simulink model "BasicSimulink"  (R2020a)
settings: configuration reference "Configuration" (kept outside this file)
PostLoadFcn:
  | if(exist('BasicSimulink_init_DB.m','file'))
  | BasicSimulink_init_DB
  | else
  | BasicSimulink_init
  | end
values from neighbouring files (symbols this model uses):
  Sim = genTurbineModelParameters(simParam,modelData)    [BasicSimulink_init.m]
undefined symbols (not defined in the file or in its folder): Const, ControllerState, OpMode
libraries: CustomBlocks_lib x1, TurbinePhysics_lib x1
settings Model: Creator=12650008  LastModifiedBy=80679
settings ConfigSetRef: SourceName=Configuration  SourceLocation=Base Workspace

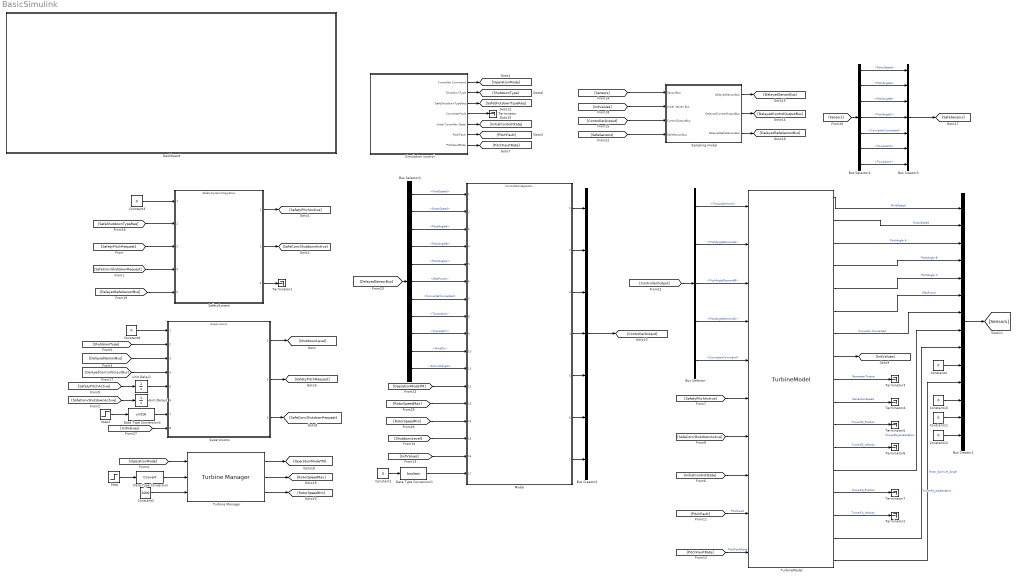
== system BasicSimulink ==
  Bus Creator1 : BusCreator  Inputs=14  OutDataTypeStr=Bus: SensorBus  NonVirtualBus=on
      settings: InheritFromInputs=off
  Bus Creator2 : BusCreator  Inputs=7  OutDataTypeStr=Bus: ControllerOutputBus  NonVirtualBus=on
      settings: InheritFromInputs=off
  Bus Creator3 : BusCreator  Inputs=7  OutDataTypeStr=Bus: SafeSensorBus  NonVirtualBus=on
      settings: InheritFromInputs=off
  Bus Selector : BusSelector  OutputSignals=TorqueDemand,PitchAngleDemandA,PitchAngleDemandB,PitchAngleDemandC,ConverterCommand
  Bus Selector1 : BusSelector  OutputSignals=WindSpeed,RotorSpeed,PitchAngleA,PitchAngleB,PitchAngleC,ElecPower,ConverterConnected,TowerAccX,TowerAccY,WindDir,AzimuthAngle
  Bus Selector2 : BusSelector  OutputSignals=RotorSpeed,PitchAngleA,PitchAngleB,PitchAngleC,ConverterConnected,TowerAccX,TowerAccY
  Constant1 : Constant  Value=0  OutDataTypeStr=boolean
  Constant{4,10..12} (4 alike) : Constant  Value=0
  Constant2 : Constant  Value=1000  OutDataTypeStr=uint16
  Constant3 : Constant  Value=0  OutDataTypeStr=boolean
  Constant6 : Constant  Value=0  OutDataTypeStr=boolean
  Dashboard : Subsystem
  Data Type Conversion : DataTypeConversion
  Data Type Conversion1 : DataTypeConversion  OutDataTypeStr=boolean
  Data Type Conversion3 : DataTypeConversion  OutDataTypeStr=uint16
  Model : ModelReference  ModelNameDialog=ControllerIntegration.slx  SimulationMode=Normal  ModelReferenceVersion=1.784
  SafetySystem : ModelReference  ModelNameDialog=SafetySystemIntegration.slx  SimulationMode=Normal  ModelReferenceVersion=1.139
  Sampling model : Subsystem
  Simulation control : Subsystem  mask{SimCase=1, VarType=NormalProduction}
      mask prompts: SimCase "Case"; VarType "Simulink:Variants:LabelComboBox"
      mask init:
      | switch (SimCase)
      |     case 1
      |         set_param(gcbh,'VarType','NormalProduction');
      |     case 2
      |         set_param(gcbh,'VarType','Startup');
      |     case 3
      |         set_param(gcbh,'VarType','Shutdown');
      |     case 4
      |         set_param(gcbh,'VarType','NoPitch');
      |     case 5
      |         set_param(gcbh,'VarType','NoTorque');
      |     case 6
      |         set_param(gcbh,'VarType','SafetySystem');
      |     case 7
      |         set_param(gcbh,'VarType','PitchRunaway');
      | end
      mask TypeOptions VarType: Scenario control/LabelModeActiveChoice
      mask DialogControl VarType Prompt: Label mode active choice:
  Step : Step  Time=3000  After=0  SampleTime=Const.Ts
  Step2 : Step  Time=30  Before=32  After=0  SampleTime=Const.Ts
  Supervisions : ModelReference  ModelNameDialog=Supervisions.slx  SimulationMode=Normal  ModelReferenceVersion=1.118
  Terminator{,1..7} (8 alike) : Terminator
  Turbine Manager : CustomBlocks_lib/Turbine Manager  SystemSampleTime=-1  Latency=0  AutoFrameSizeCalculation=off
      settings: SourceProductName=SEWPG Library
  TurbineModel : TurbinePhysics_lib/TurbineModel  Ts=Const.Ts  SimCase=6  RotAzimuthInit=0  EnableTurbulence=0  ScaleTurbulence=0.5  Seed=315  WindSpdMean=25  MeanShape=3  SineAmplitude=6  SineFrequency=0.01  RampSlope=0.01  RotorDiameter=Sim.RotorDiameter  AirDensity=Sim.AirDensity  CpData=Sim.Cp_data  CpTSR=Sim.Cp_TSR  CpPitch=Sim.Cp_pitch  dCpData=Sim.dCpdBeta  CtData=Sim.Ct_data  CtTSR=Sim.Ct_TSR  CtPitch=Sim.Ct_pitch  MaxPitch=Sim.MaxPitch  MinPitch=Sim.MinPitch  P_term=Sim.PitchSpeedGain  Acc_LimitUpper=Sim.PitchAccRateMax  Acc_LimitLower=Sim.PitchAccRateMin  MaxPitchRate=Sim.PitchModelRamp  PitchTau=Sim.PitchTau  InitialPitch=Sim.InitialPitch  PitchDelay=Sim.PitchModelDelay  SafetyPitchRate=Sim.SafetyPitchRate  Inertia=Sim.Inertia  GearRatio=Sim.GearRatio  FrictionOffset=Sim.FrictionOffset  FrictionGain=Sim.FrictionGain  DriveTrainModelSelector=Sim.DriveTrainModelSelector  MechLossTorqBp=Sim.MechLoss.TorqueBp  MechLossSpdBp=Sim.MechLoss.SpdBp  MechLossData=Sim.MechLoss.Table  BladedMechLossBp=Sim.BladedMechLossBp  BladedMechLoss=Sim.BladedMechLoss  ConverterTimeConstant=Sim.ConverterTimeConstant  ConverterConnectDelay=Sim.ConverterConnectDelay  DecayTime=Sim.ConverterDecayTime  K_comp=Sim.K_LossCompGain  LossCompMinRotSpdFactor=Sim.LossCompMinRotSpdFactor  minRotSpd=Sim.RotorSpdMin  ElEffData=Sim.ElecEff.Table  EllEffSpeedBp=Sim.ElecEff.SpdBp  ElEffPowBp=Sim.ElecEff.PowBp  BladedElecLoss=Sim.BladedElecLoss  BladedElecLossBp=Sim.BladedElecLossBp  OwnConsData=Sim.OwnCons.Table  OwnConsSpeedBp=Sim.OwnCons.SpdBp  MaxTorqueSpdSlope=Sim.MaxTorqueSpdSlope  MaxTorqueLim=Sim.MaxTorqueLim  MinTorqueSpdSlope=Sim.MinTorqueSpdSlope  MinTorqueLim=Sim.MinTorqueLim  MaxSpeedLim=Sim.MaxSpeedLim  RotorSpeedFiltFreq=Sim.RotorSpeedFiltFreq  EnableTorqueSpeedLimit=Sim.EnableTorqueSpeedLimit  twrFirstModeMass=Sim.twr.FirstModeMass  twrFirstModeLogDec=Sim.twr.FirstModeLogDec  twrFirstModeFrequencyHz=Sim.twr.FirstModeFrequencyHz  twrHeight=Sim.twr.Height
      settings: SourceProductName=SEWPG Library
  Unit Delay1 : UnitDelay  SampleTime=-1  HasFrameUpgradeWarning=on
  Unit Delay2 : UnitDelay  SampleTime=-1  HasFrameUpgradeWarning=on
  wires:
  TurbineModel/7 -> Bus Creator1/7  "Conveter Connected"
  TurbineModel/8 -> [InitValues]
  Simulation control/1(Controller Command) -> [OperationMode]
  Simulation control/2(ShutdownType) -> [ShutdownType]
  Simulation control/5(Initial Controller State) -> [InitialControlState]
  [InitialControlState] -> TurbineModel/8
  [SafetyPitchActive] -> TurbineModel/6
  [SafeConvShutdownActive] -> TurbineModel/7
  TurbineModel/9 -> Terminator3/1  "GeneratorTorque"
  TurbineModel/10 -> Terminator4/1  "GeneratorSpeed"
  TurbineModel/11 -> Terminator5/1  "TowerSS_Position"
  TurbineModel/12 -> Terminator6/1  "TowerSS_Velocity"
  [ShutdownType] -> Supervisions/2
  Constant6/1 -> Supervisions/1
  Bus Creator1/1 -> [Sensors]
  Bus Creator2/1 -> [ControllerOutput]
  [DelayedControlOutputBus] -> Supervisions/4
  Unit Delay1/1 -> Supervisions/5
  Unit Delay2/1 -> Supervisions/6
  [ControllerOutput] -> Bus Selector/1
  Bus Selector/1 -> TurbineModel/1  "<TorqueDemand>"
  Bus Selector/2 -> TurbineModel/2  "<PitchAngleDemandA>"
  Bus Selector/5 -> TurbineModel/5  "<ConverterCommand>"
  TurbineModel/1 -> Bus Creator1/1  "WindSpeed"
  TurbineModel/2 -> Bus Creator1/2  "RotorSpeed"
  TurbineModel/6 -> Bus Creator1/6  "ElecPower"
  Supervisions/3 -> [SafeConvShutdownRequest]
  Supervisions/2 -> [SafetyPitchRequest]
  SafetySystem/1 -> [SafetyPitchActive]
  SafetySystem/2 -> [SafeConvShutdownActive]
  [SafeConvShutdownActive] -> Unit Delay2/1
  [SafetyPitchActive] -> Unit Delay1/1
  Supervisions/1 -> [ShutdownLevel]
  [PitchFault] -> TurbineModel/9  "PitchFault"
  [PitchFaultRate] -> TurbineModel/10  "PitchFaultRate"
  Simulation control/6(PitchFault) -> [PitchFault]
  Simulation control/7(PitchFaultRate) -> [PitchFaultRate]
  Constant3/1 -> SafetySystem/1
  [SafeConvShutdownRequest] -> SafetySystem/4
  [SafetyPitchRequest] -> SafetySystem/3
  Simulation control/4(ConverterFault) -> Terminator/1
  Simulation control/3(SafeShutdownTypeReq) -> [SafeShutdownTypeReq]
  [SafeShutdownTypeReq] -> SafetySystem/2
  SafetySystem/3 -> Terminator1/1
  [DelayedSensorBus] -> Supervisions/3
  [DelayedSensorBus] -> Bus Selector1/1
  [Sensors] -> Sampling model/1(SensorBus)
  [InitValues] -> Sampling model/2(Initial Values Bus)
  [ControllerOutput] -> Sampling model/3(ControlOutputBus)
  Sampling model/1(DelayedSensorBus) -> [DelayedSensorBus]
  Sampling model/2(DelayedControlOutputBus) -> [DelayedControlOutputBus]
  TurbineModel/13 -> Bus Creator1/8  "TowerSS_acceleration"
  Bus Creator3/1 -> [SafeSensors]
  Bus Selector2/7 -> Bus Creator3/7  "<TowerAccY>"
  Bus Selector2/6 -> Bus Creator3/6  "<TowerAccX>"
  Bus Selector2/5 -> Bus Creator3/5  "<ConverterConnected>"
  Bus Selector2/4 -> Bus Creator3/4  "<PitchAngleC>"
  Bus Selector2/3 -> Bus Creator3/3  "<PitchAngleB>"
  Bus Selector2/2 -> Bus Creator3/2  "<PitchAngleA>"
  Bus Selector2/1 -> Bus Creator3/1  "<RotorSpeed>"
  [DelayedSafeSensorBus] -> SafetySystem/5
  [Sensors] -> Bus Selector2/1
  [SafeSensors] -> Sampling model/4(SafeSensorBus)
  Sampling model/3(DelayedSafeSensorBus) -> [DelayedSafeSensorBus]
  Step/1 -> Data Type Conversion/1
  Turbine Manager/1 -> [OperationModeTM]
  Turbine Manager/2 -> [RotorSpeedMax]
  Turbine Manager/3 -> [RotorSpeedMin]
  Data Type Conversion/1 -> Turbine Manager/2
  Step2/1 -> Data Type Conversion3/1
  Constant2/1 -> Turbine Manager/3
  Model/1 -> Bus Creator2/1
  Model/2 -> Bus Creator2/2
  Model/3 -> Bus Creator2/3
  Model/4 -> Bus Creator2/4
  Model/5 -> Bus Creator2/5
  Model/6 -> Bus Creator2/6
  Model/7 -> Bus Creator2/7
  [InitValues] -> Model/16
  [ShutdownLevel] -> Model/15
  [RotorSpeedMin] -> Model/14
  [OperationModeTM] -> Model/12
  [RotorSpeedMax] -> Model/13
  Constant12/1 -> Bus Creator1/14
  Constant11/1 -> Bus Creator1/13
  Constant10/1 -> Bus Creator1/12
  Data Type Conversion3/1 -> Supervisions/7
  [InitValues] -> Supervisions/8
  [OperationMode] -> Turbine Manager/1
  Constant1/1 -> Data Type Conversion1/1
  Data Type Conversion1/1 -> Model/17
  TurbineModel/14 -> Terminator7/1  "TowerFA_Position"
  TurbineModel/15 -> Terminator2/1  "TowerFA_Velocity"
  TurbineModel/16 -> Bus Creator1/9  "TowerFA_acceleration"
  TurbineModel/17 -> Bus Creator1/11  "Rotor_Azimuth_Angle"
  Constant4/1 -> Bus Creator1/10
  Bus Selector/3 -> TurbineModel/3  "<PitchAngleDemandB>"
  Bus Selector/4 -> TurbineModel/4  "<PitchAngleDemandC>"
  TurbineModel/3 -> Bus Creator1/3  "PitchAngle A"
  TurbineModel/4 -> Bus Creator1/4  "PitchAngle B"
  TurbineModel/5 -> Bus Creator1/5  "PitchAngle C"
  Bus Selector1/1 -> Model/1  "<WindSpeed>"
  Bus Selector1/2 -> Model/2  "<RotorSpeed>"
  Bus Selector1/3 -> Model/3  "<PitchAngleA>"
  Bus Selector1/4 -> Model/4  "<PitchAngleB>"
  Bus Selector1/5 -> Model/5  "<PitchAngleC>"
  Bus Selector1/6 -> Model/6  "<ElecPower>"
  Bus Selector1/7 -> Model/7  "<ConverterConnected>"
  Bus Selector1/8 -> Model/8  "<TowerAccX>"
  Bus Selector1/9 -> Model/9  "<TowerAccY>"
  Bus Selector1/10 -> Model/10  "<WindDir>"
  Bus Selector1/11 -> Model/11  "<AzimuthAngle>"

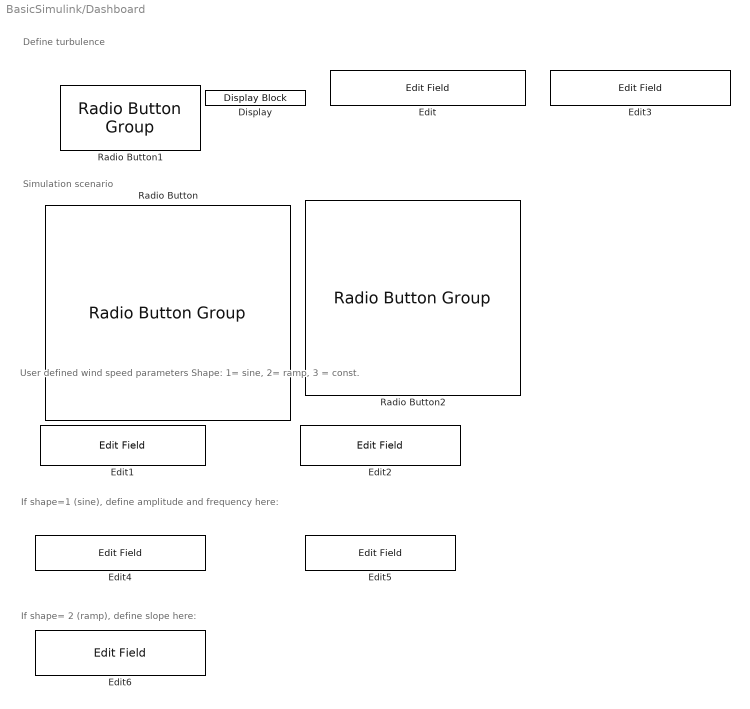
== system BasicSimulink/Dashboard ==
  note: Simulation scenario
  note: Define turbulence
  note: If shape= 2 (ramp), define slope here:
  note: If shape=1 (sine), define amplitude and frequency here:
  note: User defined wind speed parameters
      | Shape: 1= sine, 2= ramp, 3 = const.
  Display : DisplayBlock  LabelPosition=Hide  Format=Custom  Transparency=1  Layout=Fill available space  FormatString=Simulation time: %d
  Edit{,1..6} (7 alike) : EditField  ShowInitialText=on  Alignment=Center
  Radio Button : RadioButtonGroup  LabelPosition=Hide  SelectedLabel=6: User defined by parameters  ButtonGroupName=Wind Speed Control
      settings: Values={{'1: Low Wind', '2: Medium Wind', '3: High Wind', '4: Ramp mean wind speed', '5: Sinusoidal Wind Speed', '6: User defined by parameters'}, [1 2 3 4 5 6]}
  Radio Button1 : RadioButtonGroup  LabelPosition=Hide  SelectedLabel=Disabled  ButtonGroupName=Turbulence
      settings: Values={{'Disabled', 'Enabled'}, [0 1]}
  Radio Button2 : RadioButtonGroup  LabelPosition=Hide  SelectedLabel=Normal Production  ButtonGroupName=Simulation Control
      settings: Values={{'Normal Production', 'Startup', 'Shutdown (normal)', 'Shutdown (PitchFault)', 'Shutdown (Converter fault)', 'Shutdown (SafetySystem)', 'PitchRunaway'}, [1 2 3 4 5 6 7]}

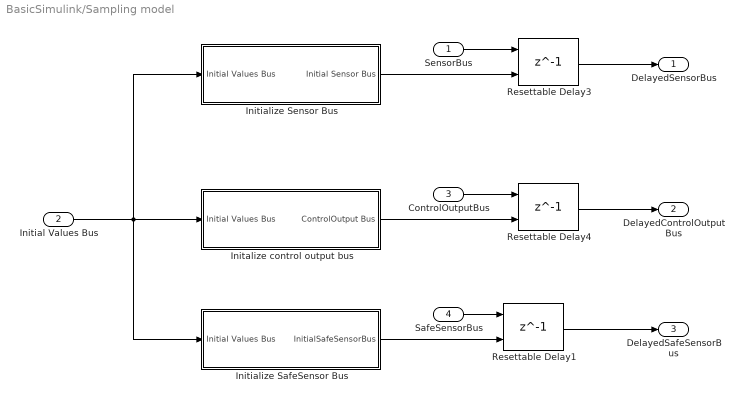
== system BasicSimulink/Sampling model ==
  SensorBus : Inport
  Initial Values Bus : Inport  Port=2
  ControlOutputBus : Inport  Port=3
  SafeSensorBus : Inport  Port=4
  Initalize control output bus : Subsystem  mask{gearratio=Sim.GearRatio}
      mask prompts: gearratio "Gear ratio"
      mask TypeOptions gearratio: GearRatio/Value
  Initialize SafeSensor Bus : Subsystem
  Initialize Sensor Bus : Subsystem
  Resettable Delay1 : Delay  DelayLength=1  InitialConditionSource=Input port  SampleTime=Const.Ts
      settings: InputPortMap=u0,p4
  Resettable Delay3 : Delay  DelayLength=1  InitialConditionSource=Input port  SampleTime=Const.Ts
      settings: InputPortMap=u0,p4
  Resettable Delay4 : Delay  DelayLength=1  InitialConditionSource=Input port  SampleTime=Const.Ts
      settings: InputPortMap=u0,p4
  DelayedSensorBus : Outport
  DelayedControlOutputBus : Outport  Port=2
  DelayedSafeSensorBus : Outport  Port=3
  wires:
  Initalize control output bus/1(ControlOutput Bus) -> Resettable Delay4/2
  Initialize Sensor Bus/1(Initial Sensor Bus) -> Resettable Delay3/2
  Resettable Delay4/1 -> DelayedControlOutputBus/1
  ControlOutputBus/1 -> Resettable Delay4/1
  Resettable Delay3/1 -> DelayedSensorBus/1
  SensorBus/1 -> Resettable Delay3/1
  Initial Values Bus/1 -> Initalize control output bus/1(Initial Values Bus), Initialize SafeSensor Bus/1(Initial Values Bus), Initialize Sensor Bus/1(Initial Values Bus)
  Initialize SafeSensor Bus/1(InitialSafeSensorBus) -> Resettable Delay1/2
  Resettable Delay1/1 -> DelayedSafeSensorBus/1
  SafeSensorBus/1 -> Resettable Delay1/1

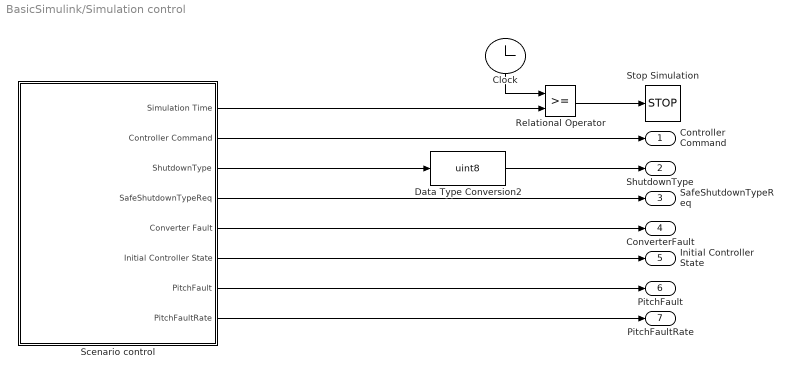
== system BasicSimulink/Simulation control ==
  Clock : Clock
  Data Type Conversion2 : DataTypeConversion  OutDataTypeStr=uint8
  Relational Operator : RelationalOperator  OutDataTypeStr=boolean  RndMeth=Simplest
  Scenario control : Subsystem  Variant=on  VariantControlMode=Label  VariantControl=Startup  LabelModeActiveChoice=NormalProduction
  Stop Simulation : Stop
  Controller Command : Outport
  ShutdownType : Outport  Port=2
  SafeShutdownTypeReq : Outport  Port=3
  ConverterFault : Outport  Port=4
  Initial Controller State : Outport  Port=5
  PitchFault : Outport  Port=6
  PitchFaultRate : Outport  Port=7
  wires:
  Clock/1 -> Relational Operator/1
  Relational Operator/1 -> Stop Simulation/1
  Scenario control/1(Simulation Time) -> Relational Operator/2
  Scenario control/4(SafeShutdownTypeReq) -> SafeShutdownTypeReq/1
  Scenario control/5(Converter Fault) -> ConverterFault/1
  Scenario control/3(ShutdownType) -> Data Type Conversion2/1
  Scenario control/6(Initial Controller State) -> Initial Controller State/1
  Scenario control/2(Controller Command) -> Controller Command/1
  Data Type Conversion2/1 -> ShutdownType/1
  Scenario control/7(PitchFault) -> PitchFault/1
  Scenario control/8(PitchFaultRate) -> PitchFaultRate/1

== system BasicSimulink/Sampling model/Initalize control output bus ==
  Initial Values Bus : Inport
  Bus Creator3 : BusCreator  Inputs=7  OutDataTypeStr=Bus: ControllerOutputBus  NonVirtualBus=on
      settings: InheritFromInputs=off
  Bus Selector2 : BusSelector  OutputSignals=RotorTorque,PitchAngle,RotorSpeed,ControllerState
  Constant : Constant  Value=ControllerState.Production  OutDataTypeStr=Enum: ControllerState
  Constant1 : Constant  Value=ControllerState.Production  OutDataTypeStr=Enum: ControllerState
  Data Type Conversion : DataTypeConversion  OutDataTypeStr=uint8
  Divide : Product  Inputs=*/
  GearRatio : Constant  Value=gearratio
  Relational Operator : RelationalOperator  Operator===  OutDataTypeStr=boolean  RndMeth=Nearest
  ControlOutput Bus : Outport
  wires:
  Bus Selector2/3 -> Bus Creator3/6  "<RotorSpeed>"
  Bus Selector2/2 -> Bus Creator3/5, Bus Creator3/4, Bus Creator3/3  "<PitchAngle>"
  Divide/1 -> Bus Creator3/2  "InitGenTorque"
  Bus Selector2/1 -> Divide/1  "<RotorTorque>"
  Relational Operator/1 -> Data Type Conversion/1  "ConverterCommand"
  Bus Creator3/1 -> ControlOutput Bus/1
  Initial Values Bus/1 -> Bus Selector2/1
  GearRatio/1 -> Divide/2
  Bus Selector2/4 -> Relational Operator/1  "<ControllerState>"
  Constant/1 -> Bus Creator3/1
  Data Type Conversion/1 -> Bus Creator3/7
  Constant1/1 -> Relational Operator/2

== system BasicSimulink/Sampling model/Initialize SafeSensor Bus ==
  note: FixMe. When correct initialization of the measurement is available.
  Initial Values Bus : Inport
  Bus Creator3 : BusCreator  Inputs=7  OutDataTypeStr=Bus: SafeSensorBus  NonVirtualBus=on
      settings: InheritFromInputs=off
  Bus Selector2 : BusSelector  OutputSignals=RotorSpeed,PitchAngle,ControllerState
  Constant : Constant  Value=0
  Constant1 : Constant  Value=0
  Constant2 : Constant  Value=ControllerState.Production  OutDataTypeStr=Enum: ControllerState
  Relational Operator : RelationalOperator  Operator===  OutDataTypeStr=boolean  RndMeth=Nearest
  InitialSafeSensorBus : Outport
  wires:
  Constant1/1 -> Bus Creator3/7  "TowerAccY"
  Constant/1 -> Bus Creator3/6  "TowerAccX"
  Relational Operator/1 -> Bus Creator3/5  "ConverterConnected"
  Bus Selector2/3 -> Relational Operator/1  "<ControllerState>"
  Bus Selector2/2 -> Bus Creator3/3, Bus Creator3/4, Bus Creator3/2  "<PitchAngle>"
  Bus Selector2/1 -> Bus Creator3/1  "<RotorSpeed>"
  Bus Creator3/1 -> InitialSafeSensorBus/1
  Initial Values Bus/1 -> Bus Selector2/1
  Constant2/1 -> Relational Operator/2

== system BasicSimulink/Sampling model/Initialize Sensor Bus ==
  Initial Values Bus : Inport
  Bus Creator3 : BusCreator  Inputs=14  OutDataTypeStr=Bus: SensorBus  NonVirtualBus=on
      settings: InheritFromInputs=off
  Bus Selector2 : BusSelector  OutputSignals=WindSpeed,RotorSpeed,PitchAngle,ControllerState
  Constant : Constant  Value=0
  Constant1 : Constant  Value=0
  Constant2 : Constant  Value=ControllerState.Production  OutDataTypeStr=Enum: ControllerState
  Relational Operator : RelationalOperator  Operator===  OutDataTypeStr=boolean  RndMeth=Nearest
  Initial Sensor Bus : Outport
  wires:
  Constant1/1 -> Bus Creator3/9, Bus Creator3/8, Bus Creator3/11, Bus Creator3/12, Bus Creator3/13, Bus Creator3/14, Bus Creator3/10
  Relational Operator/1 -> Bus Creator3/7
  Constant/1 -> Bus Creator3/6
  Bus Selector2/4 -> Relational Operator/1  "<ControllerState>"
  Bus Selector2/3 -> Bus Creator3/5, Bus Creator3/4, Bus Creator3/3  "<PitchAngle>"
  Bus Selector2/2 -> Bus Creator3/2  "<RotorSpeed>"
  Bus Selector2/1 -> Bus Creator3/1  "<WindSpeed>"
  Bus Creator3/1 -> Initial Sensor Bus/1
  Initial Values Bus/1 -> Bus Selector2/1
  Constant2/1 -> Relational Operator/2

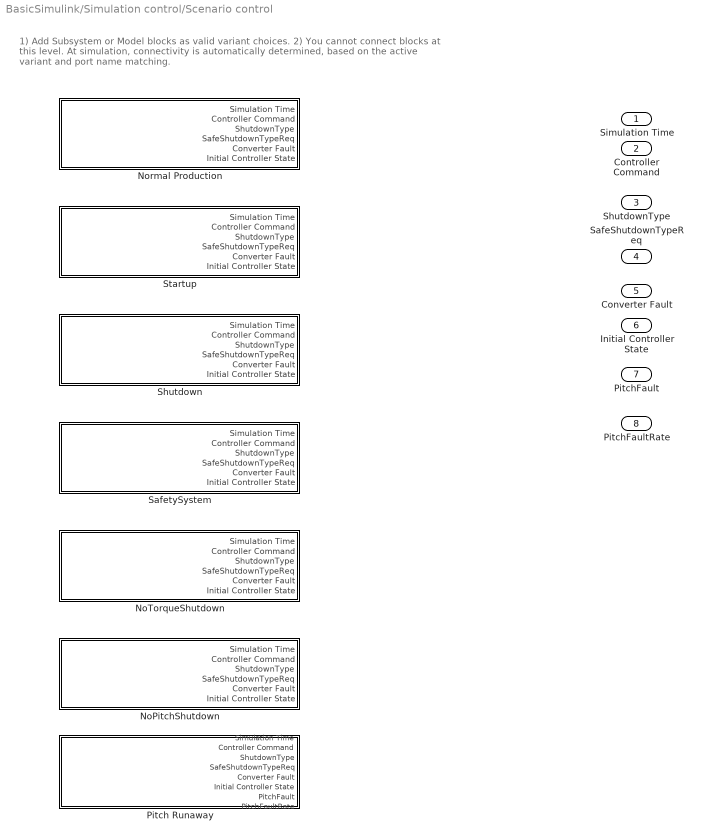
== system BasicSimulink/Simulation control/Scenario control ==
  note: 1) Add Subsystem or Model blocks as valid variant choices.
      | 2) You cannot connect blocks at this level. At simulation, connectivity is automatically
      | determined, based on the active variant and port name matching.
  NoPitchShutdown : Subsystem  VariantControl=NoPitch
  NoTorqueShutdown : Subsystem  VariantControl=NoTorque
  Normal Production : Subsystem  VariantControl=NormalProduction
  Pitch Runaway : Subsystem  VariantControl=PitchRunaway
  SafetySystem : Subsystem  VariantControl=SafetySystem
  Shutdown : Subsystem  VariantControl=Shutdown
  Startup : Subsystem  VariantControl=Startup
  Simulation Time : Outport
  Controller Command : Outport  Port=2
  ShutdownType : Outport  Port=3
  SafeShutdownTypeReq : Outport  Port=4
  Converter Fault : Outport  Port=5
  Initial Controller State : Outport  Port=6
  PitchFault : Outport  Port=7
  PitchFaultRate : Outport  Port=8

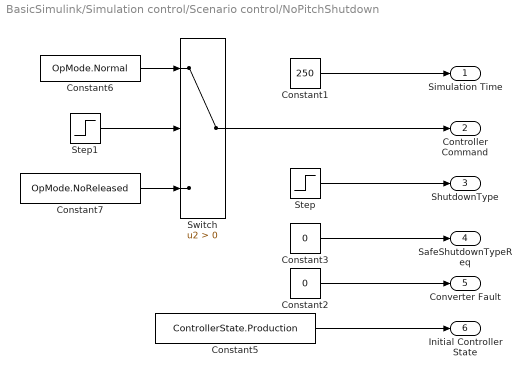
== system BasicSimulink/Simulation control/Scenario control/NoPitchShutdown ==
  Constant1 : Constant  Value=250
  Constant2 : Constant  Value=0
  Constant3 : Constant  Value=0
  Constant5 : Constant  Value=ControllerState.Production
  Constant6 : Constant  Value=OpMode.Normal
  Constant7 : Constant  Value=OpMode.NoReleased
  Step : Step  Time=25  After=3  SampleTime=0
  Step1 : Step  Time=25  Before=1  After=0  SampleTime=0
  Switch : Switch  Criteria=u2 > Threshold
  Simulation Time : Outport
  Controller Command : Outport  Port=2
  ShutdownType : Outport  Port=3
  SafeShutdownTypeReq : Outport  Port=4
  Converter Fault : Outport  Port=5
  Initial Controller State : Outport  Port=6
  wires:
  Switch/1 -> Controller Command/1
  Constant1/1 -> Simulation Time/1
  Constant3/1 -> SafeShutdownTypeReq/1
  Constant2/1 -> Converter Fault/1
  Constant5/1 -> Initial Controller State/1
  Step/1 -> ShutdownType/1
  Step1/1 -> Switch/2
  Constant6/1 -> Switch/1
  Constant7/1 -> Switch/3

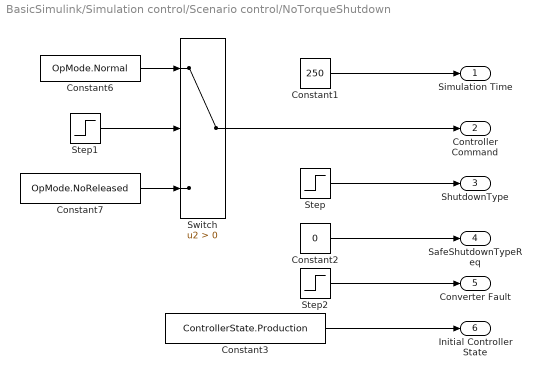
== system BasicSimulink/Simulation control/Scenario control/NoTorqueShutdown ==
  Constant1 : Constant  Value=250
  Constant2 : Constant  Value=0
  Constant3 : Constant  Value=ControllerState.Production
  Constant6 : Constant  Value=OpMode.Normal
  Constant7 : Constant  Value=OpMode.NoReleased
  Step : Step  Time=25  After=2  SampleTime=0
  Step1 : Step  Time=25  Before=1  After=0  SampleTime=0
  Step2 : Step  Time=25  SampleTime=0
  Switch : Switch  Criteria=u2 > Threshold
  Simulation Time : Outport
  Controller Command : Outport  Port=2
  ShutdownType : Outport  Port=3
  SafeShutdownTypeReq : Outport  Port=4
  Converter Fault : Outport  Port=5
  Initial Controller State : Outport  Port=6
  wires:
  Switch/1 -> Controller Command/1
  Constant1/1 -> Simulation Time/1
  Constant2/1 -> SafeShutdownTypeReq/1
  Step2/1 -> Converter Fault/1
  Constant3/1 -> Initial Controller State/1
  Step/1 -> ShutdownType/1
  Step1/1 -> Switch/2
  Constant6/1 -> Switch/1
  Constant7/1 -> Switch/3

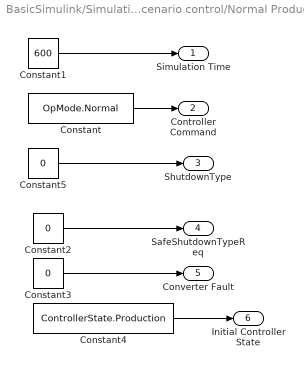
== system BasicSimulink/Simulation control/Scenario control/Normal Production ==
  Constant : Constant  Value=OpMode.Normal
  Constant1 : Constant  Value=600
  Constant2 : Constant  Value=0
  Constant3 : Constant  Value=0
  Constant4 : Constant  Value=ControllerState.Production
  Constant5 : Constant  Value=0
  Simulation Time : Outport
  Controller Command : Outport  Port=2
  ShutdownType : Outport  Port=3
  SafeShutdownTypeReq : Outport  Port=4
  Converter Fault : Outport  Port=5
  Initial Controller State : Outport  Port=6
  wires:
  Constant2/1 -> SafeShutdownTypeReq/1
  Constant3/1 -> Converter Fault/1
  Constant4/1 -> Initial Controller State/1
  Constant1/1 -> Simulation Time/1
  Constant5/1 -> ShutdownType/1
  Constant/1 -> Controller Command/1

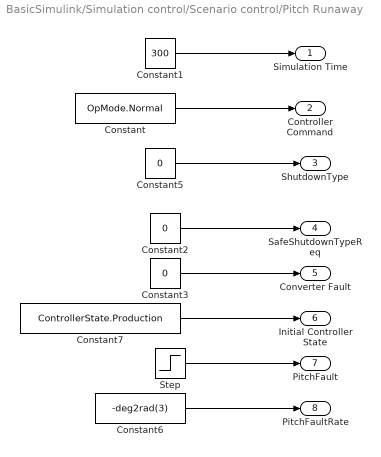
== system BasicSimulink/Simulation control/Scenario control/Pitch Runaway ==
  Constant : Constant  Value=OpMode.Normal
  Constant1 : Constant  Value=300
  Constant2 : Constant  Value=0
  Constant3 : Constant  Value=0
  Constant5 : Constant  Value=0
  Constant6 : Constant  Value=-deg2rad(3)
  Constant7 : Constant  Value=ControllerState.Production
  Step : Step  Time=30  After=2  SampleTime=Const.Ts
  Simulation Time : Outport
  Controller Command : Outport  Port=2
  ShutdownType : Outport  Port=3
  SafeShutdownTypeReq : Outport  Port=4
  Converter Fault : Outport  Port=5
  Initial Controller State : Outport  Port=6
  PitchFault : Outport  Port=7
  PitchFaultRate : Outport  Port=8
  wires:
  Constant/1 -> Controller Command/1
  Constant2/1 -> SafeShutdownTypeReq/1
  Constant3/1 -> Converter Fault/1
  Constant7/1 -> Initial Controller State/1
  Constant1/1 -> Simulation Time/1
  Constant5/1 -> ShutdownType/1
  Step/1 -> PitchFault/1
  Constant6/1 -> PitchFaultRate/1

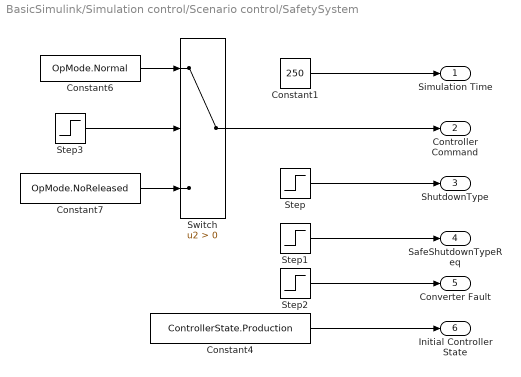
== system BasicSimulink/Simulation control/Scenario control/SafetySystem ==
  Constant1 : Constant  Value=250
  Constant4 : Constant  Value=ControllerState.Production
  Constant6 : Constant  Value=OpMode.Normal
  Constant7 : Constant  Value=OpMode.NoReleased
  Step : Step  Time=25  After=0  SampleTime=0
  Step1 : Step  Time=25  After=4  SampleTime=0
  Step2 : Step  Time=25  SampleTime=0
  Step3 : Step  Time=25  Before=1  After=0  SampleTime=0
  Switch : Switch  Criteria=u2 > Threshold
  Simulation Time : Outport
  Controller Command : Outport  Port=2
  ShutdownType : Outport  Port=3
  SafeShutdownTypeReq : Outport  Port=4
  Converter Fault : Outport  Port=5
  Initial Controller State : Outport  Port=6
  wires:
  Constant1/1 -> Simulation Time/1
  Step1/1 -> SafeShutdownTypeReq/1
  Step2/1 -> Converter Fault/1
  Constant4/1 -> Initial Controller State/1
  Step/1 -> ShutdownType/1
  Step3/1 -> Switch/2
  Constant6/1 -> Switch/1
  Switch/1 -> Controller Command/1
  Constant7/1 -> Switch/3

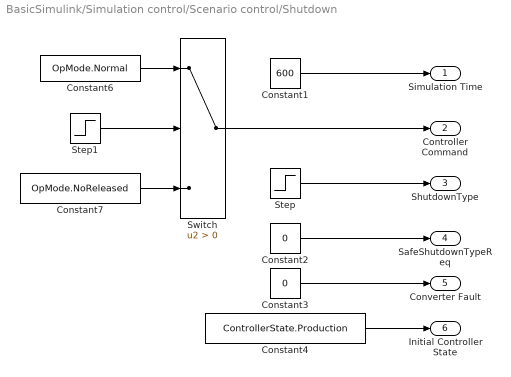
== system BasicSimulink/Simulation control/Scenario control/Shutdown ==
  Constant1 : Constant  Value=600
  Constant2 : Constant  Value=0
  Constant3 : Constant  Value=0
  Constant4 : Constant  Value=ControllerState.Production
  Constant6 : Constant  Value=OpMode.Normal
  Constant7 : Constant  Value=OpMode.NoReleased
  Step : Step  Time=200  SampleTime=0
  Step1 : Step  Time=25  Before=1  After=0  SampleTime=0
  Switch : Switch  Criteria=u2 > Threshold
  Simulation Time : Outport
  Controller Command : Outport  Port=2
  ShutdownType : Outport  Port=3
  SafeShutdownTypeReq : Outport  Port=4
  Converter Fault : Outport  Port=5
  Initial Controller State : Outport  Port=6
  wires:
  Constant1/1 -> Simulation Time/1
  Constant2/1 -> SafeShutdownTypeReq/1
  Constant3/1 -> Converter Fault/1
  Constant4/1 -> Initial Controller State/1
  Step/1 -> ShutdownType/1
  Switch/1 -> Controller Command/1
  Step1/1 -> Switch/2
  Constant7/1 -> Switch/3
  Constant6/1 -> Switch/1

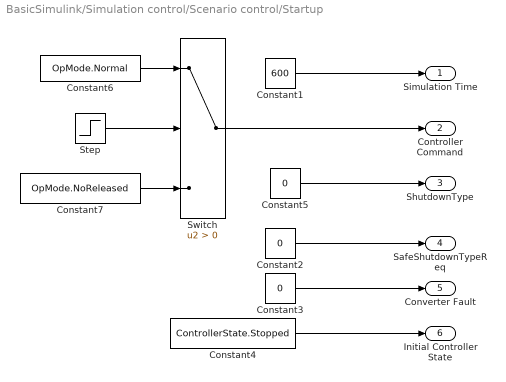
== system BasicSimulink/Simulation control/Scenario control/Startup ==
  Constant1 : Constant  Value=600
  Constant2 : Constant  Value=0
  Constant3 : Constant  Value=0
  Constant4 : Constant  Value=ControllerState.Stopped
  Constant5 : Constant  Value=0
  Constant6 : Constant  Value=OpMode.Normal
  Constant7 : Constant  Value=OpMode.NoReleased
  Step : Step  Time=25  SampleTime=0
  Switch : Switch  Criteria=u2 > Threshold
  Simulation Time : Outport
  Controller Command : Outport  Port=2
  ShutdownType : Outport  Port=3
  SafeShutdownTypeReq : Outport  Port=4
  Converter Fault : Outport  Port=5
  Initial Controller State : Outport  Port=6
  wires:
  Constant1/1 -> Simulation Time/1
  Constant2/1 -> SafeShutdownTypeReq/1
  Constant3/1 -> Converter Fault/1
  Constant4/1 -> Initial Controller State/1
  Constant5/1 -> ShutdownType/1
  Switch/1 -> Controller Command/1
  Step/1 -> Switch/2
  Constant6/1 -> Switch/1
  Constant7/1 -> Switch/3
